simulink model "t3_4"  (R2017b)
settings: Solver=VariableStepAuto  StartTime=0.0  StopTime=100  RelTol=1e-3
libraries: simulink x1
settings Model: Creator=zxy19  LastModifiedBy=zxy19

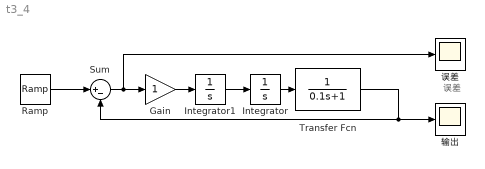
== system t3_4 ==
  note: 误差
  Gain : Gain
  Integrator : Integrator
  Integrator1 : Integrator
  Ramp : simulink/Sources/Ramp  slope=1  start=0  X0=0
  Sum : Sum  Inputs=|+-
  Transfer Fcn : TransferFcn  Denominator=[0.1 1]
  误差 : Scope
  输出 : Scope
  wires:
  Ramp/1 -> Sum/1
  Sum/1 -> 误差/1, Gain/1
  Gain/1 -> Integrator1/1
  Integrator/1 -> Transfer Fcn/1
  Transfer Fcn/1 -> 输出/1, Sum/2
  Integrator1/1 -> Integrator/1
